simulink model "Commander_Stabilizer_Qdrone_serial"  (R2019a)
settings: Solver=ode2  StartTime=0.0  StopTime=inf  FixedStep=0.001  RelTol=1e-3  EnableMultiTasking=on
InitFcn:
  | set_param(gcs, 'ZoomFactor','FitSystem')
model workspace (MAT data in the model file):
  target_system = 1
undefined symbols (not defined in the file or in its folder): HIL, qc_get_step_size
libraries: quarc_library x53, simulink x24, simulink_extras x4
(part 1 of 4)
settings Model: SimulationMode=external  ExtModeTrigDuration=10000  Creator=dmadill  LastModifiedBy=user
settings SolverCC: PositivePriorityOrder=on
settings DataIOCC: LimitDataPoints=on  SaveFormat=Array  ReturnWorkspaceOutputs=off
settings OptimizationCC: LifeSpan=inf
settings DebuggingCC: SolverPrmCheckMsg=warning  SFUnexpectedBacktrackingDiag=warning  SFNoUnconditionalDefaultTransitionDiag=warning  SFExecutionAtInitializationDiag=none  ArithmeticOperatorsInVariantConditions=warning
settings HardwareCC: ProdBitPerLong=64  ProdLargestAtomicFloat=None  ProdHWDeviceType=Intel->x86-64
settings ModelReferenceCC: PropagateSignalLabelsOutOfModel=off
settings SFSimCC: SimUseLocalCustomCode=off
settings RTWCC: SystemTargetFile=quarc_linux_x64.tlc  TemplateMakefile=quarc_linux_x64_tmf  Description=QUARC Linux x64 Target  RTWUseLocalCustomCode=off
settings CodeAppCC: StateflowObjectComments=on
settings STFCustomTargetCC: TargetLibSuffix=.a  TargetPreCompLibLocation=C:\PROGRA~3\QUARC\lib\2019a\LINUX_~1\release  ConcurrentExecutionCompliant=on  SystemTargetFile=quarc_linux_x64.tlc
settings GRTTargetCC: TargetLibSuffix=.a  TargetPreCompLibLocation=C:\PROGRA~3\QUARC\lib\2019a\LINUX_~1\release  TargetLangStandard=C89/C90 (ANSI)  ParMdlRefBuildCompliant=off  CompOptLevelCompliant=off  CombineOutputUpdateFcns=off  MatFileLogging=off  CPPClassGenCompliant=off  GRTInterface=on  UseToolchainInfoCompliant=off  ExtMode=on  ExtModeMexFile=quarc_comm  ExtModeMexArgs='-w -d /tmp -uri %u -IP_address tcpip://192.168.1.157:18000', 'tcpip://192.168.1.25:17001?retries=10'
settings ConfigComp: CovMetricSettings=dw  CovHtmlReporting=on  CovSaveCumulativeToWorkspaceVar=on  CovSaveSingleToWorkspaceVar=on  CovExternalEMLEnable=off  CovSFcnEnable=off

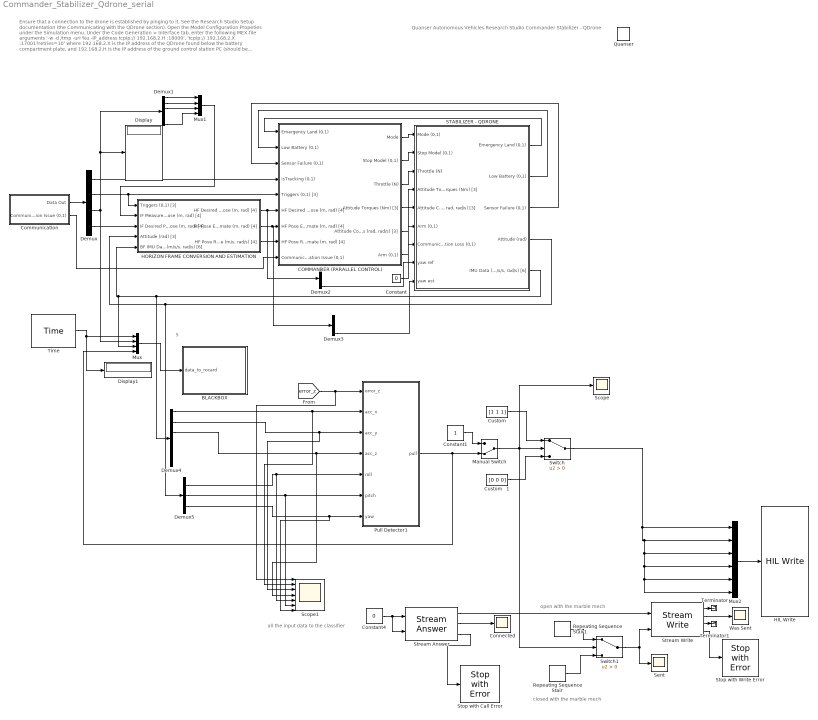
== system Commander_Stabilizer_Qdrone_serial ==
  note: all the input data to the classifier
  note: closed with the marble mech
  note: open with the marble mech
  note: Quanser Autonomous Vehicles Research Studio
      | Commander Stabilizer - QDrone
  note: Ensure that a connection to the drone is established by pinging to it. See the Research Studio Setup documentation (the Communicating with the QDrone section).
      | Open the Model Configuration Propeties under the Simulation menu.
      | Under the Code Generation > Interface tab, enter the following MEX-file arguments
      | '-w -d /tmp -uri %u -IP_address tcpip:// 192.168.2.H :18000', 'tcpip:// 192.168.2.X :17001?retries=10'
      | where 192.168.2.X is the IP address of the QDrone found below the battery compartment plate, and 192.168.2.H is the IP address of the ground control station PC (should be 192.168.2.5 by default).
      |
      | Under the QUARC menu, click on Build .
      |
      | Ensure that the Mission_Server_QDrone_Position_Control.slx model is running. If not, this model will stop immediately upon running. Click on Start under the QUARC menu.
      |
      | Ensure that the drone behaves as expected (see the steps in the Mission_Server_QDrone_Position_Control.slx model)
      | This model will automatically stop when the QDrone lands.
  note: 5
  "   Custom   " : Constant  Value=[1 1 1]
  "   Custom   1" : Constant  Value=[0 0 0]
  BLACKBOX : Subsystem
  COMMANDER (PARALLEL CONTROL) : Subsystem
  Communication : Subsystem
  Connected : Scope
  Constant : Constant  Value=0
  Constant1 : Constant
  Constant4 : Constant  Value=0
  Demux : Demux  Outputs=[1 3 6 4]
  Demux1 : Demux  Outputs=6
  Demux2 : Demux
  Demux3 : Demux
  Demux4 : Demux  Outputs=6
  Demux5 : Demux  Outputs=3
  Display : Display
  Display1 : Display
  HIL Write : quarc_library/Data Acquisition/Generic/Immediate I//O/HIL Write  object_name=HIL-1  analog_channels=[]  pwm_channels=[]  digital_channels=[5:7 9:23]  other_channels=[]  sample_time=-1  active=off  vector_input=on
      settings: SourceProductName=The database C:\Users\user\AppData\Roaming\MathWorks\MATLAB\R2017a\slblocks_master.db is locked, or a table in the database is locked. (database is locked)
  HORIZON FRAME CONVERSION AND ESTIMATION : Subsystem
  Manual Switch : ManualSwitch  CurrentSetting=0
  Mux : Mux  Inputs=[1 6 6 1]
  Mux1 : Mux
  Mux2 : Mux  Inputs=6
  Pull Detector1 : Subsystem
  Quanser : quarc_library/Logos/Quanser
  Repeating Sequence Stair : simulink/Sources/Repeating Sequence Stair  OutValues=[255 255 1 7 3 30 0 0 0 0 214].'  tsamp=-1  OutMin=[0]  OutMax=[]  OutDataTypeStr=fixdt(0,8,0)  OutputDataTypeScalingMode=Specify via dialog  OutDataType=fixdt(0,8,0)  ConRadixGroup=Best Precision: Vector-wise  OutScaling=[]
  Repeating Sequence Stair1 : simulink/Sources/Repeating Sequence Stair  OutValues=[255 255 1 7 3 30 32 3 0 0 179].'  tsamp=-1  OutMin=[0]  OutMax=[]  OutDataTypeStr=fixdt(0,8,0)  OutputDataTypeScalingMode=Specify via dialog  OutDataType=fixdt(0,8,0)  ConRadixGroup=Best Precision: Vector-wise  OutScaling=[]
  "STABILIZER - QDRONE " : Subsystem
  Scope : Scope
  Scope1 : Scope  NumInputPorts=7
  Sent : Scope
  Stop with Call Error : quarc_library/Sinks/Error Handling/Stop with Error  message_type=Interpret input as error code  message=Error occurred
      settings: SourceProductName=QUARC Targets
  Stop with Write Error : quarc_library/Sinks/Error Handling/Stop with Error  message_type=Interpret input as error code  message=Error occurred
      settings: SourceProductName=QUARC Targets
  Stream Answer : quarc_library/Communications/Intermediate/Stream Answer  uri_source=Specify via dialog (do not evaluate)  uri=serial://localhost:1?sndsize='16',baud='9600',word='8'  apply_uri_to_all_configs=on  send_buffer_size=128  receive_buffer_size=128  byte_order=little endian (Intel - LSB first)  sample_time=qc_get_step_size  active=off
      settings: AttributesFormatString="\"serial://localhost:1?sndsize='16',baud='9600',word='8'\""  SourceProductName=QUARC Targets
  Stream Write : quarc_library/Communications/Intermediate/Stream Write  optimization=Minimizing latency  send_dims=off
      settings: SourceProductName=QUARC Targets
  Switch : Switch  Criteria=u2 > Threshold
  Switch1 : Switch  Criteria=u2 > Threshold
  Terminator : Terminator
  Terminator1 : Terminator
  Time : quarc_library/Sources/Time/Time  time_source=Process CPU time  sample_time=qc_get_step_size
  Was Sent : Scope
  wires:
  COMMANDER (PARALLEL CONTROL)/2(Stop Model (0,1)) -> "STABILIZER - QDRONE "/2(Stop Model (0,1))
  "STABILIZER - QDRONE "/1(Emergency Land (0,1)) -> COMMANDER (PARALLEL CONTROL)/1(Emergency Land (0,1))
  COMMANDER (PARALLEL CONTROL)/4(Attitude Torques (Nm) [3]) -> "STABILIZER - QDRONE "/4(Attitude Torques (Nm) [3])
  Communication/1(Data Out) -> Demux/1
  Demux/2 -> COMMANDER (PARALLEL CONTROL)/5(Triggers (0,1) [3]), HORIZON FRAME CONVERSION AND ESTIMATION/1(Triggers (0,1) [3])
  "STABILIZER - QDRONE "/2(Low Battery (0,1)) -> COMMANDER (PARALLEL CONTROL)/2(Low Battery (0,1))
  "STABILIZER - QDRONE "/3(Sensor Failure (0,1)) -> COMMANDER (PARALLEL CONTROL)/3(Sensor Failure (0,1))
  COMMANDER (PARALLEL CONTROL)/6(Arm (0,1)) -> "STABILIZER - QDRONE "/6(Arm (0,1))
  COMMANDER (PARALLEL CONTROL)/3(Throttle (N)) -> "STABILIZER - QDRONE "/3(Throttle (N))
  Constant/1 -> "STABILIZER - QDRONE "/7(Communication Loss (0,1))
  COMMANDER (PARALLEL CONTROL)/5("Attitude Commands (rad, rad/s) [3]") -> "STABILIZER - QDRONE "/5("Attitude Commands (rad, rad, rad/s) [3]")
  COMMANDER (PARALLEL CONTROL)/1(Mode) -> "STABILIZER - QDRONE "/1(Mode (0,1))
  Communication/2(Communication Issue (0,1)) -> COMMANDER (PARALLEL CONTROL)/9(Communication Issue (0,1))
  "STABILIZER - QDRONE "/4(Attitude (rad)) -> Demux5/1, HORIZON FRAME CONVERSION AND ESTIMATION/4(Attitude (rad) [3])
  "STABILIZER - QDRONE "/5("IMU Data (m/s/s, rad/s) [6]") -> Demux4/1, Mux/3, HORIZON FRAME CONVERSION AND ESTIMATION/5("BF IMU Data (m/s/s, rad/s) [6]")
  HORIZON FRAME CONVERSION AND ESTIMATION/3("HF Pose Rate Estimate (m/s, rad/s) [4]") -> COMMANDER (PARALLEL CONTROL)/8("HF Pose Rate Estimate (m, rad) [4]")
  Demux/1 -> COMMANDER (PARALLEL CONTROL)/4(isTracking (0,1))
  Demux/4 -> HORIZON FRAME CONVERSION AND ESTIMATION/3("IF Desired Pose (m, rad) [4]")
  Demux/3 -> Demux1/1, Display/1, Mux/2
  Mux1/1 -> HORIZON FRAME CONVERSION AND ESTIMATION/2("IF Measured Pose (m, rad) [4]")
  Demux1/3 -> Mux1/3
  Demux1/6 -> Mux1/4
  Demux1/2 -> Mux1/2
  Demux1/1 -> Mux1/1
  Mux/1 -> BLACKBOX/1("data_to_rocard ")
  Time/1 -> Display1/1, Mux/1
  Demux2/4 -> "STABILIZER - QDRONE "/8(yaw ref)
  HORIZON FRAME CONVERSION AND ESTIMATION/1("HF Desired Pose (m, rad) [4]") -> Demux2/1, COMMANDER (PARALLEL CONTROL)/6("HF Desired Pose (m, rad) [4]")
  Demux3/4 -> "STABILIZER - QDRONE "/9(yaw est)
  HORIZON FRAME CONVERSION AND ESTIMATION/2("HF Pose Estimate (m, rad) [4]") -> Demux3/1, COMMANDER (PARALLEL CONTROL)/7("HF Pose Estimate (m, rad) [4]")
  Demux4/1 -> Pull Detector1/2(acc_x), Scope1/2
  Demux4/2 -> Pull Detector1/3(acc_y), Scope1/3
  Demux4/3 -> Pull Detector1/4(acc_z), Scope1/4
  [error_z] -> Scope1/1, Pull Detector1/1(error_z)
  Demux5/1 -> Pull Detector1/5(roll), Scope1/5
  Demux5/2 -> Pull Detector1/6(pitch), Scope1/6
  Demux5/3 -> Scope1/7, Pull Detector1/7(yaw)
  Mux2/1 -> HIL Write/1
  Switch/1 -> Mux2/6, Mux2/5, Mux2/4, Mux2/3, Mux2/2, Mux2/1
  Pull Detector1/1(pull) -> Mux/4, Manual Switch/2
  Manual Switch/1 -> Switch1/2, Switch/2, Scope/1
  "   Custom   "/1 -> Switch/1
  "   Custom   1"/1 -> Switch/3
  Constant1/1 -> Manual Switch/1
  Stream Write/4 -> Stop with Write Error/1
  Stream Answer/2 -> Connected/1
  Stream Write/3 -> Terminator1/1
  Stream Write/2 -> Was Sent/1
  Stream Answer/3 -> Stop with Call Error/1
  Stream Answer/1 -> Stream Write/1
  Switch1/1 -> Stream Write/2, Sent/1
  Constant4/1 -> Stream Answer/1, Stream Answer/2
  Stream Write/1 -> Terminator/1
  Repeating Sequence Stair1/1 -> Switch1/1
  Repeating Sequence Stair/1 -> Switch1/3

== system Commander_Stabilizer_Qdrone_serial/BLACKBOX ==
  "data_to_rocard " : Inport
  To Host File : quarc_library/Sinks/To Host/To Host File  file_name=saved_data/%m/record_data_%{date}_%{time}.mat  variable_name=optitack_imu_data  decimation=1  sample_time=-1  file_format=MAT-file v.5  options=No header or footer  append=off  final_file_name=saved_data/Commander_Stabilizer_Qdrone_serial/record_data_04-Apr-2021_22-18-28.mat  bitrate=2000000
  wires:
  "data_to_rocard "/1 -> To Host File/1

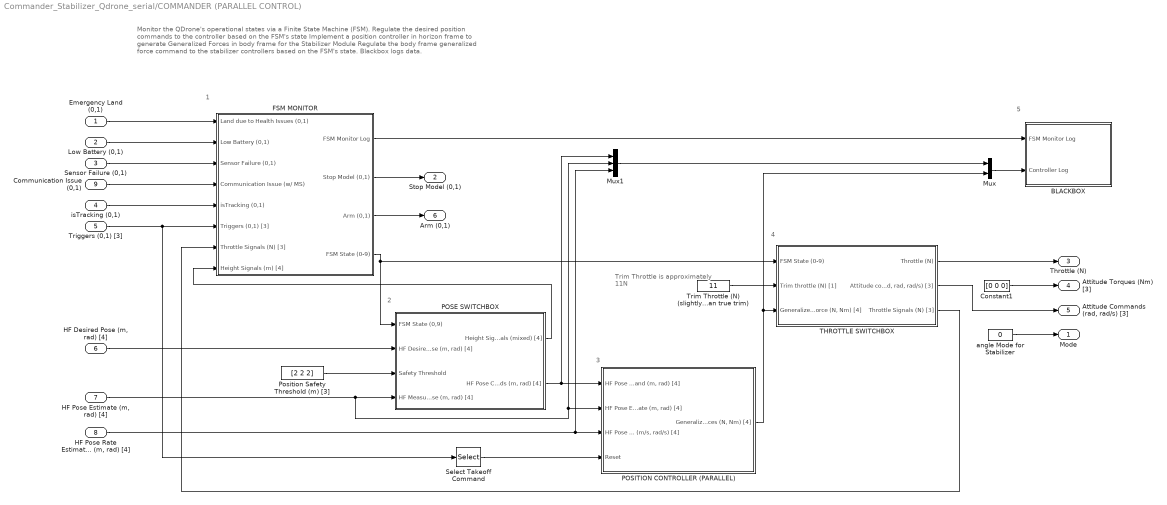
== system Commander_Stabilizer_Qdrone_serial/COMMANDER (PARALLEL CONTROL) ==
  note: 5
  note: 4
  note: 3
  note: 2
  note: 1
  note: Monitor the QDrone's operational states via a Finite State Machine (FSM).
      | Regulate the desired position commands to the controller based on the FSM's state
      | Implement a position controller in horizon frame to generate Generalized Forces in body frame for the Stabilizer Module
      | Regulate the body frame generalized force command to the stabilizer controllers based on the FSM's state.
      | Blackbox logs data.
  note: Trim Throttle is approximately 11N
  Emergency Land (0,1) : Inport
  Low Battery (0,1) : Inport  Port=2
  Sensor Failure (0,1) : Inport  Port=3
  isTracking (0,1) : Inport  Port=4
  Triggers (0,1) [3] : Inport  Port=5
  "HF Desired Pose (m, rad) [4]" : Inport  Port=6
  "HF Pose Estimate (m, rad) [4]" : Inport  Port=7
  "HF Pose Rate Estimate (m, rad) [4]" : Inport  Port=8
  Communication Issue (0,1) : Inport  Port=9
  BLACKBOX : Subsystem
  Constant1 : Constant  Value=[0 0 0]
  FSM MONITOR : Subsystem
  Mux : Mux  Inputs=2
  Mux1 : Mux  Inputs=3
  POSE SWITCHBOX : Subsystem
  POSITION CONTROLLER (PARALLEL) : Subsystem
  Position Safety Threshold (m) [3] : Constant  Value=[2 2 2]
  Select Takeoff Command : Selector  InputPortWidth=3  IndexOptions=Index vector (dialog)  Indices=[2]  OutputSizes=1
  "THROTTLE SWITCHBOX " : Subsystem
  Trim Throttle (N) (slightly lower than true trim) : Constant  Value=11
  angle Mode for Stabilizer : Constant  Value=0
  Mode : Outport
  Stop Model (0,1) : Outport  Port=2
  Throttle (N) : Outport  Port=3
  Attitude Torques (Nm) [3] : Outport  Port=4
  "Attitude Commands (rad, rad/s) [3]" : Outport  Port=5
  Arm (0,1) : Outport  Port=6
  wires:
  FSM MONITOR/1(FSM Monitor Log) -> BLACKBOX/1(FSM Monitor Log)
  FSM MONITOR/2(Stop Model (0,1)) -> Stop Model (0,1)/1
  FSM MONITOR/3(Arm (0,1)) -> Arm (0,1)/1
  Emergency Land (0,1)/1 -> FSM MONITOR/1(Land due to Health Issues (0,1))
  Low Battery (0,1)/1 -> FSM MONITOR/2(Low Battery (0,1))
  Sensor Failure (0,1)/1 -> FSM MONITOR/3(Sensor Failure (0,1))
  Communication Issue (0,1)/1 -> FSM MONITOR/4(Communication Issue (w/ MS))
  isTracking (0,1)/1 -> FSM MONITOR/5(isTracking (0,1))
  Select Takeoff Command/1 -> POSITION CONTROLLER (PARALLEL)/4(Reset)
  angle Mode for Stabilizer/1 -> Mode/1
  "HF Pose Estimate (m, rad) [4]"/1 -> Mux1/2, POSITION CONTROLLER (PARALLEL)/2("HF Pose Estimate (m, rad) [4]"), POSE SWITCHBOX/4("HF Measured Pose (m, rad) [4]")
  "HF Pose Rate Estimate (m, rad) [4]"/1 -> Mux1/3, POSITION CONTROLLER (PARALLEL)/3("HF Pose Rate (m/s, rad/s) [4]")
  Trim Throttle (N) (slightly lower than true trim)/1 -> "THROTTLE SWITCHBOX "/2(Trim throttle (N) [1])
  POSITION CONTROLLER (PARALLEL)/1("Generalized Forces (N, Nm) [4]") -> Mux/2, "THROTTLE SWITCHBOX "/3("Generalized Force (N, Nm) [4]")
  "HF Desired Pose (m, rad) [4]"/1 -> POSE SWITCHBOX/2("HF Desired Pose (m, rad) [4]")
  Position Safety Threshold (m) [3]/1 -> POSE SWITCHBOX/3(Safety Threshold)
  FSM MONITOR/4(FSM State (0-9)) -> POSE SWITCHBOX/1(FSM State (0,9)), "THROTTLE SWITCHBOX "/1(FSM State (0-9))
  "THROTTLE SWITCHBOX "/1(Throttle (N)) -> Throttle (N)/1
  POSE SWITCHBOX/1(Height Signals (mixed) [4]) -> FSM MONITOR/8(Height Signals (m) [4])
  "THROTTLE SWITCHBOX "/3(Throttle Signals (N) [3]) -> FSM MONITOR/7(Throttle Signals (N) [3])
  Triggers (0,1) [3]/1 -> FSM MONITOR/6(Triggers (0,1) [3]), Select Takeoff Command/1
  Mux/1 -> BLACKBOX/2(Controller Log)
  POSE SWITCHBOX/2("HF Pose Commands (m, rad) [4]") -> Mux1/1, POSITION CONTROLLER (PARALLEL)/1("HF Pose Command (m, rad) [4]")
  Mux1/1 -> Mux/1
  Constant1/1 -> Attitude Torques (Nm) [3]/1
  "THROTTLE SWITCHBOX "/2("Attitude commands (rad, rad, rad/s) [3]") -> "Attitude Commands (rad, rad/s) [3]"/1

== system Commander_Stabilizer_Qdrone_serial/Communication ==
  note: Argument (- IP_address ) is set at the MEX-file arguments found at Model Configuration Properties > Code Generation > Interface
      |
      | Format:
      | tcpip://192.168.2.H:18000
      | where H is the last digits of your ground station's IP address (use ipconfig in a command prompt to find it out).
  Constant : Constant
  Detect Communication Loss : Subsystem
  Display : Display
  Memory : Memory  InheritSampleTime=on  LinearizeMemory=on  LinearizeAsDelay=on
  Model Argument : quarc_library/Sources/Signals/Model Argument  argument_name=IP_address  has_value=on  data_type_mode=Specify via dialog  data_type=char  max_length=80  variable_size=off
      settings: AttributesFormatString=(-%<argument_name>)  SourceProductName=QUARC Targets
  Select Timestamp received and send back immediately (for calculating loopback time) : Selector  InputPortWidth=15  IndexOptions=Index vector (dialog)  Indices=[15]  OutputSizes=1
  Select the rest of the data : Selector  InputPortWidth=15  IndexOptions=Index vector (dialog)  Indices=[1:14]  OutputSizes=1
  Stream Client : quarc_library/Communications/Basic/Stream Client  uri_source=External input port  uri=tcpip://192.168.2.3:18669  apply_uri_to_all_configs=on  send_buffer_size=1460  receive_buffer_size=1460  byte_order=little endian (Intel - LSB first)  optimization=Minimum latency  send_options=Send most recent data  receive_options=Receive most recent data  default_value=zeros(1,15)  sample_time=qc_get_step_size  active=off  implementation=Use blocking I/O in a separate thread  send_fifo_size=1000  receive_fifo_size=1000  send_priority=0  receive_priority=0  send_dimensions=off  receive_dimensions=off  max_dimensions=-1  data_type=Inherited via back propagation  type_expr=BusObject
  String Display : quarc_library/Strings/String Display  alignment=center  display_mode=Single line  sample_time=-1
      settings: SourceProductName=QUARC Targets
  Terminator1 : Terminator
  Terminator2 : Terminator
  Data Out : Outport
  Communication Issue (0,1) : Outport  Port=2
  wires:
  Stream Client/5 -> Terminator2/1
  Model Argument/1 -> Stream Client/3, String Display/1
  Constant/1 -> Stream Client/2
  Stream Client/3 -> Terminator1/1
  Stream Client/4 -> Detect Communication Loss/3(Data Out), Select Timestamp received and send back immediately (for calculating loopback time)/1, Select the rest of the data/1
  Memory/1 -> Stream Client/1
  Stream Client/1 -> Detect Communication Loss/1(State)
  Stream Client/2 -> Detect Communication Loss/2(Error)
  Detect Communication Loss/1(Communication Issue) -> Communication Issue (0,1)/1
  Select the rest of the data/1 -> Data Out/1
  Select Timestamp received and send back immediately (for calculating loopback time)/1 -> Display/1, Memory/1

== system Commander_Stabilizer_Qdrone_serial/HORIZON FRAME CONVERSION AND ESTIMATION ==
  note: IF => Inertial Frame
      | BF => Body Frame
      | HF => Horizon Frame
  note: 6
  note: 5
  note: 4
  note: 3
  note: 2
  note: 1
  note: Steps:
      |
      | Estimate the Yaw Angle from the gyroscopic yaw rate signal and the localization yaw correction signal.
      | Use this yaw estimate, along with the roll/pitch estimates from the stabilizer to calculate the rotation matrices that convert data from the Body and Inertial Frames to the Horizon frame, where position control takes place
      | Transform Body Frame Net Accelerations (from accelerometer) to Horizon Frame Vehicle Accelerations
      | Transform Inertial Frame Desired and Measured Positions to the Horizon Frame Pose Commands and Estimates respectively
      | Calculate the Pose Rate Estimates
      | Saturate and Rate Limit the IF Desired Pose based on workspace limitations
  Triggers (0,1) [3] : Inport
  "IF Measured Pose (m, rad) [4]" : Inport  Port=2
  "IF Desired Pose (m, rad) [4]" : Inport  Port=3
  Attitude (rad) [3] : Inport  Port=4
  "BF IMU Data (m/s/s, rad/s) [6]" : Inport  Port=5
  Calculate Rotation Matrices : Subsystem
  Estimate Yaw Angle : Subsystem
  Pitch : Selector  InputPortWidth=3  IndexOptions=Index vector (dialog)  Indices=[2]  OutputSizes=1
  Pose Rate Estimation : Subsystem
  Rate Limiter : RateLimiter  RisingSlewLimit=[2 2 3 2]  FallingSlewLimit=[-2 -2 -3 -2]  SampleTimeMode=inherited  InitialCondition=[0 0 0 0]
  Roll : Selector  InputPortWidth=3  IndexOptions=Index vector (dialog)  Indices=[1]  OutputSizes=1
  Saturation : Saturate  UpperLimit=[2.5 2.5 3 Inf]  LowerLimit=[-2.5 -2.5 0 -Inf]
  Select Gyro Yaw Rate (rad/s) : Selector  InputPortWidth=6  IndexOptions=Index vector (dialog)  Indices=[6]  OutputSizes=1
  Select Linear Acceleration : Selector  InputPortWidth=6  IndexOptions=Index vector (dialog)  Indices=[1 2 3]  OutputSizes=1
  Select Takeoff Command : Selector  InputPortWidth=3  IndexOptions=Index vector (dialog)  Indices=[2]  OutputSizes=1
  Select Yaw Estimate : Selector  InputPortWidth=4  IndexOptions=Index vector (dialog)  Indices=4  OutputSizes=1
  Transform from Body Frame to Horizon Frame : Subsystem
  Transform from Inertial Frame to Horizon Frame : Subsystem
  "HF Desired Pose (m, rad) [4]" : Outport
  "HF Pose Estimate (m, rad) [4]" : Outport  Port=2
  "HF Pose Rate Estimate (m/s, rad/s) [4]" : Outport  Port=3
  wires:
  "BF IMU Data (m/s/s, rad/s) [6]"/1 -> Select Linear Acceleration/1, Select Gyro Yaw Rate (rad/s)/1
  Select Gyro Yaw Rate (rad/s)/1 -> Estimate Yaw Angle/1(Yaw Rate (rad/s)), Pose Rate Estimation/3(Yaw Rate (rad/s))  "Gyroscope Yaw Rate (rad/s)"
  "IF Measured Pose (m, rad) [4]"/1 -> Transform from Inertial Frame to Horizon Frame/4("IF Pose Measurement (m, rad) [4]"), Select Yaw Estimate/1
  Estimate Yaw Angle/1(Yaw Estimate (rad)) -> Transform from Inertial Frame to Horizon Frame/3(Yaw Estimate), Calculate Rotation Matrices/3(Yaw Estimate (rad))
  Select Yaw Estimate/1 -> Estimate Yaw Angle/2(Yaw Correction (rad))
  Triggers (0,1) [3]/1 -> Select Takeoff Command/1
  Attitude (rad) [3]/1 -> Pitch/1, Roll/1
  Roll/1 -> Calculate Rotation Matrices/1(" Roll Estimate (rad)")
  Pitch/1 -> Calculate Rotation Matrices/2(Pitch Estimate (rad))
  Pose Rate Estimation/1("HF Pose Rate Estimate (m/s, rad/s) [4]") -> "HF Pose Rate Estimate (m/s, rad/s) [4]"/1
  Transform from Inertial Frame to Horizon Frame/1("HF Pose Estimate (m, rad) [4]") -> "HF Pose Estimate (m, rad) [4]"/1, Pose Rate Estimation/2("HF Pose Measurement (m, rad) [4]")
  Calculate Rotation Matrices/2(HF_R_IF) -> Transform from Inertial Frame to Horizon Frame/1(HF_R_IF)
  "IF Desired Pose (m, rad) [4]"/1 -> Saturation/1
  Transform from Inertial Frame to Horizon Frame/2("HF Pose Command (m, rad) [4]") -> "HF Desired Pose (m, rad) [4]"/1
  Calculate Rotation Matrices/1(HF_R_BF) -> Transform from Body Frame to Horizon Frame/1(HF_R_BF)
  Select Linear Acceleration/1 -> Transform from Body Frame to Horizon Frame/2(BF Net Acceleration (m/s/s) [3])  "BF Net Acceleration"
  Transform from Body Frame to Horizon Frame/1(HF Vehicle Acceleration (m/s/s) [3]) -> Pose Rate Estimation/1(HF Vehicle Acceleration (m/s/s) [3])
  Select Takeoff Command/1 -> Estimate Yaw Angle/3(Reset), Pose Rate Estimation/4(Reset)  "Reset Condition"
  Rate Limiter/1 -> Transform from Inertial Frame to Horizon Frame/2("IF Pose Command (m, rad) [4]")
  Saturation/1 -> Rate Limiter/1

== system Commander_Stabilizer_Qdrone_serial/Pull Detector1 ==
  error_z : Inport
  acc_x : Inport  Port=2
  acc_y : Inport  Port=3
  acc_z : Inport  Port=4
  roll : Inport  Port=5
  pitch : Inport  Port=6
  yaw : Inport  Port=7
  Constant : Constant  Value=50  OutDataTypeStr=single
  MATLAB Function : MATLAB Function  TreatAsAtomicUnit=on
  MATLAB Function1 : MATLAB Function  TreatAsAtomicUnit=on
  Scope4 : Scope  NumInputPorts=3
  pull : Outport  VectorParamsAs1DForOutWhenUnconnected=on
  wires:
  yaw/1 -> MATLAB Function/7(yaw)
  roll/1 -> MATLAB Function/5(roll)
  Constant/1 -> MATLAB Function1/2(threshold)
  acc_x/1 -> MATLAB Function/2(acc_x)
  acc_y/1 -> MATLAB Function/3(acc_y)
  MATLAB Function/1(detection_output) -> MATLAB Function1/1(u), Scope4/1
  acc_z/1 -> MATLAB Function/4(acc_z)
  pitch/1 -> MATLAB Function/6(pitch)
  error_z/1 -> Scope4/3, MATLAB Function/1(error_z)
  MATLAB Function1/1(y) -> Scope4/2, pull/1

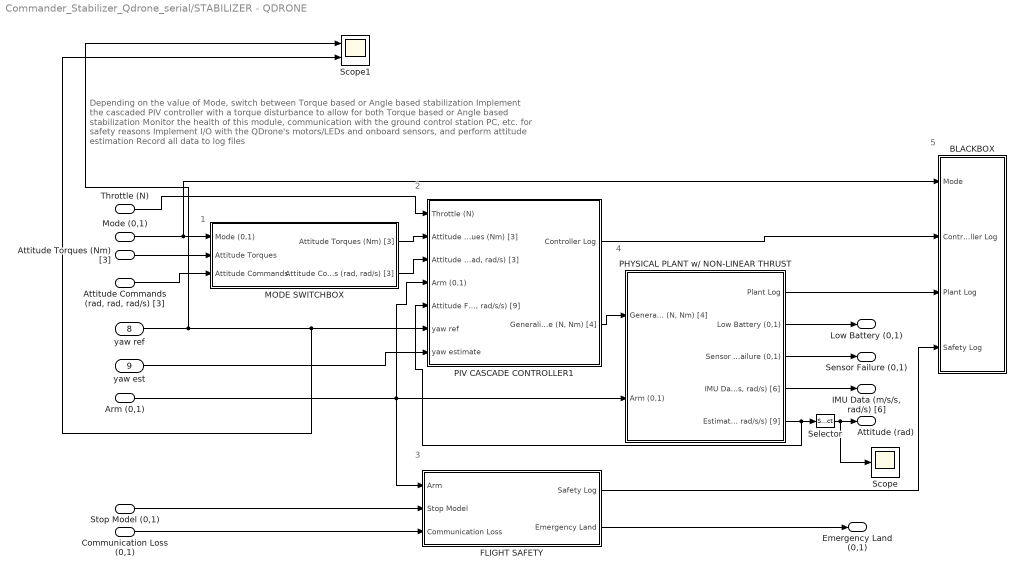
== system Commander_Stabilizer_Qdrone_serial/STABILIZER - QDRONE  ==
  note: 5
  note: 4
  note: 3
  note: 2
  note: 1
  note: Depending on the value of Mode, switch between Torque based or Angle based stabilization
      | Implement the cascaded PIV controller with a torque disturbance to allow for both Torque based or Angle based stabilization
      | Monitor the health of this module, communication with the ground control station PC, etc. for safety reasons
      | Implement I/O with the QDrone's motors/LEDs and onboard sensors, and perform attitude estimation
      | Record all data to log files
  Mode (0,1) : Inport
  Stop Model (0,1) : Inport  Port=2
  Throttle (N) : Inport  Port=3
  Attitude Torques (Nm) [3] : Inport  Port=4
  "Attitude Commands (rad, rad, rad/s) [3]" : Inport  Port=5
  Arm (0,1) : Inport  Port=6
  Communication Loss (0,1) : Inport  Port=7
  yaw ref : Inport  Port=8
  yaw est : Inport  Port=9
  BLACKBOX : Subsystem
  FLIGHT SAFETY : Subsystem
  MODE SWITCHBOX : Subsystem
  PHYSICAL PLANT w/ NON-LINEAR THRUST : Subsystem
  PIV CASCADE CONTROLLER1 : Subsystem
  Scope : Scope
  Scope1 : Scope  NumInputPorts=2
  Selector : Selector  InputPortWidth=9  IndexOptions=Index vector (dialog)  Indices=[1:3]  OutputSizes=1
  Emergency Land (0,1) : Outport
  Low Battery (0,1) : Outport  Port=2
  Sensor Failure (0,1) : Outport  Port=3
  Attitude (rad) : Outport  Port=4
  "IMU Data (m/s/s, rad/s) [6]" : Outport  Port=5
  wires:
  PIV CASCADE CONTROLLER1/1(Controller Log) -> BLACKBOX/2(Controller Log)
  Attitude Torques (Nm) [3]/1 -> MODE SWITCHBOX/2(Attitude Torques)
  PHYSICAL PLANT w/ NON-LINEAR THRUST/1(Plant Log) -> BLACKBOX/3(Plant Log)
  FLIGHT SAFETY/1(Safety Log) -> BLACKBOX/4(Safety Log)
  PHYSICAL PLANT w/ NON-LINEAR THRUST/5("Estimated Attitude (rad, rad/s, rad/s/s) [9]") -> PIV CASCADE CONTROLLER1/5("Attitude Feedback (rad, rad/s, rad/s/s) [9]"), Selector/1
  FLIGHT SAFETY/2(Emergency Land) -> Emergency Land (0,1)/1
  PIV CASCADE CONTROLLER1/2("Generalized Force (N, Nm) [4]") -> PHYSICAL PLANT w/ NON-LINEAR THRUST/1("Generalized Force (N, Nm) [4]")
  PHYSICAL PLANT w/ NON-LINEAR THRUST/2(Low Battery (0,1)) -> Low Battery (0,1)/1
  Stop Model (0,1)/1 -> FLIGHT SAFETY/2(Stop Model)
  Arm (0,1)/1 -> PIV CASCADE CONTROLLER1/4(Arm (0,1)), PHYSICAL PLANT w/ NON-LINEAR THRUST/2(Arm (0,1)), FLIGHT SAFETY/1(Arm)
  Communication Loss (0,1)/1 -> FLIGHT SAFETY/3(Communication Loss)
  PHYSICAL PLANT w/ NON-LINEAR THRUST/3(Sensor Failure (0,1)) -> Sensor Failure (0,1)/1
  PHYSICAL PLANT w/ NON-LINEAR THRUST/4("IMU Data (m/s/s, rad/s) [6]") -> "IMU Data (m/s/s, rad/s) [6]"/1
  Throttle (N)/1 -> PIV CASCADE CONTROLLER1/1(Throttle (N))
  "Attitude Commands (rad, rad, rad/s) [3]"/1 -> MODE SWITCHBOX/3(Attitude Commands)
  Mode (0,1)/1 -> BLACKBOX/1(Mode), MODE SWITCHBOX/1(Mode (0,1))
  MODE SWITCHBOX/2("Attitude Commands (rad, rad/s) [3]") -> PIV CASCADE CONTROLLER1/3("Attitude Commands (rad, rad, rad/s) [3]")
  MODE SWITCHBOX/1(Attitude Torques (Nm) [3]) -> PIV CASCADE CONTROLLER1/2(Attitude Torques (Nm) [3])
  Selector/1 -> Scope/1, Attitude (rad)/1
  yaw est/1 -> PIV CASCADE CONTROLLER1/7("yaw estimate ")
  yaw ref/1 -> Scope1/2, PIV CASCADE CONTROLLER1/6("yaw ref "), Scope1/1

== system Commander_Stabilizer_Qdrone_serial/COMMANDER (PARALLEL CONTROL)/BLACKBOX ==
  FSM Monitor Log : Inport
  Controller Log : Inport  Port=2
  Mux : Mux  Inputs=2
  To Host File : quarc_library/Sinks/To Host/To Host File  file_name=saved_data/%m/Commander_%{date}_%{time}.mat  variable_name=commander_data  decimation=1  sample_time=-1  file_format=MAT-file v.5  options=No header or footer  append=off  final_file_name=saved_data/Commander_Stabilizer_Qdrone_serial/Commander_04-Apr-2021_22-18-28.mat  bitrate=2000000
  wires:
  Mux/1 -> To Host File/1
  FSM Monitor Log/1 -> Mux/1
  Controller Log/1 -> Mux/2

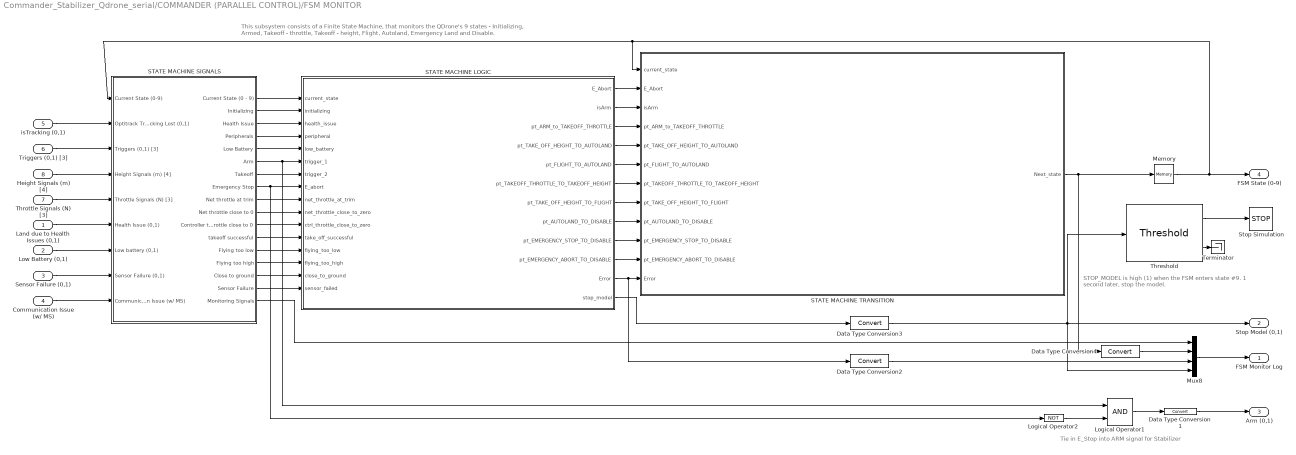
== system Commander_Stabilizer_Qdrone_serial/COMMANDER (PARALLEL CONTROL)/FSM MONITOR ==
  note: This subsystem consists of a Finite State Machine, that monitors the QDrone's 9 states - Initializing, Armed, Takeoff - throttle, Takeoff - height, Flight, Autoland, Emergency Land and Disable.
  note: Tie in E_Stop into ARM signal for Stabilizer
  note: STOP_MODEL is high (1) when the FSM enters state #9.
      | 1 second later, stop the model.
  Land due to Health Issues (0,1) : Inport
  Low Battery (0,1) : Inport  Port=2
  Sensor Failure (0,1) : Inport  Port=3
  Communication Issue (w/ MS) : Inport  Port=4
  isTracking (0,1) : Inport  Port=5
  Triggers (0,1) [3] : Inport  Port=6
  Throttle Signals (N) [3] : Inport  Port=7
  Height Signals (m) [4] : Inport  Port=8
  Data Type Conversion{1..4} (4 alike) : DataTypeConversion
  Logical Operator1 : Logic  AllPortsSameDT=off  OutDataTypeStr=boolean
  Logical Operator2 : Logic  Operator=NOT  AllPortsSameDT=off  OutDataTypeStr=boolean
  Memory : Memory  InitialCondition=1
  Mux8 : Mux  Inputs=[17 1 1 1]
  STATE MACHINE LOGIC : MATLAB Function  TreatAsAtomicUnit=on
  STATE MACHINE SIGNALS : Subsystem
  STATE MACHINE TRANSITION : MATLAB Function  TreatAsAtomicUnit=on
  Stop Simulation : Stop
  Terminator : Terminator
  Threshold : quarc_library/Discontinuities/Threshold  operator=>=  param_src=Specify via dialog  threshold=0.5  duration=1
      settings: SourceProductName=QUARC Targets
  FSM Monitor Log : Outport
  Stop Model (0,1) : Outport  Port=2
  Arm (0,1) : Outport  Port=3
  FSM State (0-9) : Outport  Port=4
  wires:
  STATE MACHINE LOGIC/1(E_Abort) -> STATE MACHINE TRANSITION/2(E_Abort)
  STATE MACHINE LOGIC/11(Error) -> STATE MACHINE TRANSITION/12(Error), Data Type Conversion2/1
  STATE MACHINE LOGIC/6(pt_TAKEOFF_THROTTLE_TO_TAKEOFF_HEIGHT) -> STATE MACHINE TRANSITION/7(pt_TAKEOFF_THROTTLE_TO_TAKEOFF_HEIGHT)
  STATE MACHINE LOGIC/7(pt_TAKE_OFF_HEIGHT_TO_FLIGHT) -> STATE MACHINE TRANSITION/8(pt_TAKE_OFF_HEIGHT_TO_FLIGHT)
  STATE MACHINE LOGIC/8(pt_AUTOLAND_TO_DISABLE) -> STATE MACHINE TRANSITION/9(pt_AUTOLAND_TO_DISABLE)
  STATE MACHINE LOGIC/9(pt_EMERGENCY_STOP_TO_DISABLE) -> STATE MACHINE TRANSITION/10(pt_EMERGENCY_STOP_TO_DISABLE)
  STATE MACHINE LOGIC/10(pt_EMERGENCY_ABORT_TO_DISABLE) -> STATE MACHINE TRANSITION/11(pt_EMERGENCY_ABORT_TO_DISABLE)
  STATE MACHINE SIGNALS/2(Initializing) -> STATE MACHINE LOGIC/2(initializing)
  STATE MACHINE SIGNALS/3(Health Issue) -> STATE MACHINE LOGIC/3(health_issue)
  STATE MACHINE SIGNALS/4(Peripherals) -> STATE MACHINE LOGIC/4(peripheral)
  STATE MACHINE SIGNALS/5(Low Battery) -> STATE MACHINE LOGIC/5(low_battery)
  STATE MACHINE SIGNALS/7(Takeoff) -> STATE MACHINE LOGIC/7(trigger_2)
  STATE MACHINE SIGNALS/9(Net throttle at trim) -> STATE MACHINE LOGIC/9(net_throttle_at_trim)
  STATE MACHINE SIGNALS/10(Net throttle close to 0) -> STATE MACHINE LOGIC/10(net_throttle_close_to_zero)
  STATE MACHINE SIGNALS/11(Controller throttle close to 0) -> STATE MACHINE LOGIC/11(ctrl_throttle_close_to_zero)
  STATE MACHINE SIGNALS/12(takeoff successful) -> STATE MACHINE LOGIC/12(take_off_successful)
  STATE MACHINE SIGNALS/13(Flying too low) -> STATE MACHINE LOGIC/13(flying_too_low)
  STATE MACHINE SIGNALS/14(Flying too high) -> STATE MACHINE LOGIC/14(flying_too_high)
  STATE MACHINE SIGNALS/15(Close to ground) -> STATE MACHINE LOGIC/15(close_to_ground)
  STATE MACHINE TRANSITION/1(Next_state) -> Data Type Conversion4/1, Memory/1
  Mux8/1 -> FSM Monitor Log/1
  STATE MACHINE SIGNALS/1("Current State (0 - 9)  ") -> STATE MACHINE LOGIC/1(current_state)
  STATE MACHINE SIGNALS/16("  Sensor Failure") -> STATE MACHINE LOGIC/16(sensor_failed)
  STATE MACHINE SIGNALS/17(Monitoring Signals) -> Mux8/1
  Sensor Failure (0,1)/1 -> STATE MACHINE SIGNALS/8(Sensor Failure (0,1))
  Low Battery (0,1)/1 -> STATE MACHINE SIGNALS/7(Low battery (0,1))
  Land due to Health Issues (0,1)/1 -> STATE MACHINE SIGNALS/6("Health Issue (0,1)  ")
  Data Type Conversion1/1 -> Arm (0,1)/1
  Logical Operator1/1 -> Data Type Conversion1/1
  STATE MACHINE SIGNALS/8(Emergency Stop) -> Logical Operator2/1, STATE MACHINE LOGIC/8(E_abort)
  Logical Operator2/1 -> Logical Operator1/2
  STATE MACHINE SIGNALS/6(Arm) -> Logical Operator1/1, STATE MACHINE LOGIC/6(trigger_1)
  Triggers (0,1) [3]/1 -> STATE MACHINE SIGNALS/3(Triggers (0,1) [3])
  Communication Issue (w/ MS)/1 -> STATE MACHINE SIGNALS/9(Communication Issue (w/ MS))
  isTracking (0,1)/1 -> STATE MACHINE SIGNALS/2("Optitrack Tracking Lost (0,1)  ")
  Data Type Conversion2/1 -> Mux8/3
  Data Type Conversion4/1 -> Mux8/2
  Throttle Signals (N) [3]/1 -> STATE MACHINE SIGNALS/5(Throttle Signals (N) [3])
  Height Signals (m) [4]/1 -> STATE MACHINE SIGNALS/4(Height Signals (m) [4])
  Threshold/2 -> Terminator/1
  Data Type Conversion3/1 -> Threshold/1, Stop Model (0,1)/1, Mux8/4
  Threshold/1 -> Stop Simulation/1
  Memory/1 -> FSM State (0-9)/1, STATE MACHINE TRANSITION/1(current_state), STATE MACHINE SIGNALS/1(Current State (0-9))
  STATE MACHINE LOGIC/2(isArm) -> STATE MACHINE TRANSITION/3(isArm)
  STATE MACHINE LOGIC/3(pt_ARM_to_TAKEOFF_THROTTLE) -> STATE MACHINE TRANSITION/4(pt_ARM_to_TAKEOFF_THROTTLE)
  STATE MACHINE LOGIC/4(pt_TAKE_OFF_HEIGHT_TO_AUTOLAND) -> STATE MACHINE TRANSITION/5(pt_TAKE_OFF_HEIGHT_TO_AUTOLAND)
  STATE MACHINE LOGIC/5(pt_FLIGHT_TO_AUTOLAND) -> STATE MACHINE TRANSITION/6(pt_FLIGHT_TO_AUTOLAND)
  STATE MACHINE LOGIC/12(stop_model) -> Data Type Conversion3/1

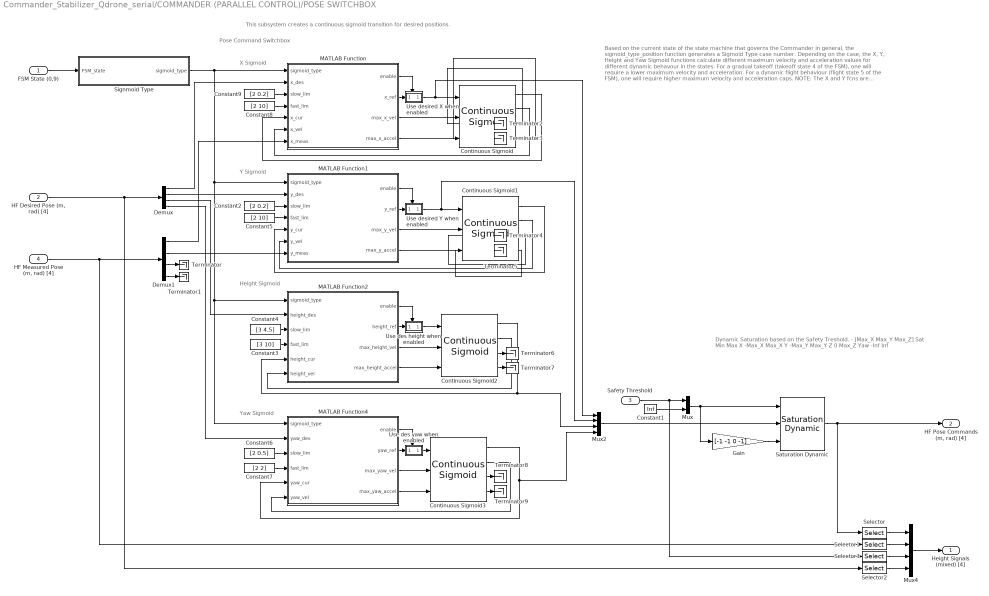
== system Commander_Stabilizer_Qdrone_serial/COMMANDER (PARALLEL CONTROL)/POSE SWITCHBOX ==
  note: Dynamic Saturation based on the Safety Treshold. - [Max_X Max_Y Max_Z]
      |
      | Sat Min Max
      | X -Max_X Max_X
      | Y -Max_Y Max_Y
      | Z 0 Max_Z
      | Yaw -Inf Inf
  note: Based on the current state of the state machine that governs the Commander in general,
      | the sigmoid_type_position function generates a Sigmoid Type case number. Depending on
      | the case, the X, Y, Height and Yaw Sigmoid functions calculate different maximum velocity
      | and acceleration values for different dynamic behavour in the states.
      |
      | For a gradual takeoff (takeoff state 4 of the FSM), one will require a lower maximum velocity
      | and acceleration. For a dynamic flight behaviour (flight state 5 of the FSM), one will require
      | higher maximum velocity and acceleration caps.
      |
      | NOTE: The X and Y fcns are logically identical due to the generally symmetric X and Y behaviour.
      | The Z and Yaw fcns are different.
  note: This subsystem creates a continuous sigmoid transition for desired positions.
  note: Height Sigmoid
  note: Pose Command Switchbox
  note: X Sigmoid
  note: Yaw Sigmoid
  note: Y Sigmoid
  FSM State (0,9) : Inport
  "HF Desired Pose (m, rad) [4]" : Inport  Port=2
  Safety Threshold : Inport  Port=3
  "HF Measured Pose (m, rad) [4]" : Inport  Port=4
  Constant1 : Constant  Value=Inf
  Constant2 : Constant  Value=[2 0.2]
  Constant3 : Constant  Value=[3 10]
  Constant4 : Constant  Value=[3 4.5]
  Constant5 : Constant  Value=[2 10]
  Constant6 : Constant  Value=[2 0.5]
  Constant7 : Constant  Value=[2 2]
  Constant8 : Constant  Value=[2 10]
  Constant9 : Constant  Value=[2 0.2]
  Continuous Sigmoid{,1..3} (4 alike) : quarc_library/Sources/Sigmoids/Continuous Sigmoid  params_source=External (input ports)  max_velocity=2  max_acceleration=10  initial_position=0  initial_velocity=0  hold_off=0.5  input_sample_time=-1  output_sample_time=qc_get_step_size
      settings: SourceProductName=QUARC Targets
  Demux : Demux
  Demux1 : Demux
  Gain : Gain  Gain=[-1 -1 0 -1]
  MATLAB Function : MATLAB Function  TreatAsAtomicUnit=on
  MATLAB Function1 : MATLAB Function  TreatAsAtomicUnit=on
  MATLAB Function2 : MATLAB Function  TreatAsAtomicUnit=on
  MATLAB Function4 : MATLAB Function  TreatAsAtomicUnit=on
  Mux : Mux  Inputs=2
  Mux2 : Mux
  Mux4 : Mux
  Saturation Dynamic : simulink/Discontinuities/Saturation Dynamic  OutMin=[]  OutMax=[]  OutDataTypeStr=Inherit: Same as second input  OutDataType=fixdt(1, 16)  OutScaling=2^-10  DoSatur=off
  Selector : Selector  InputPortWidth=4  IndexOptions=Index vector (dialog)  Indices=[3]  OutputSizes=1
  Selector1 : Selector  InputPortWidth=4  IndexOptions=Index vector (dialog)  Indices=[3]  OutputSizes=1
  Selector2 : Selector  InputPortWidth=4  IndexOptions=Index vector (dialog)  Indices=[3]  OutputSizes=1
  Selector3 : Selector  InputPortWidth=3  IndexOptions=Index vector (dialog)  Indices=[3]  OutputSizes=1
  Signmoid Type : MATLAB Function  TreatAsAtomicUnit=on
  Terminator{,1..9} (10 alike) : Terminator
  Use des height when enabled : Subsystem  TreatAsAtomicUnit=on
  Use des yaw when enabled : Subsystem  TreatAsAtomicUnit=on
  Use desired X when enabled : Subsystem  TreatAsAtomicUnit=on
  Use desired Y when enabled : Subsystem  TreatAsAtomicUnit=on
  Height Signals (mixed) [4] : Outport
  "HF Pose Commands (m, rad) [4]" : Outport  Port=2
  wires:
  Selector/1 -> Mux4/1
  Selector1/1 -> Mux4/2
  Selector2/1 -> Mux4/4
  Selector3/1 -> Mux4/3
  Safety Threshold/1 -> Mux/1, Selector3/1
  Mux/1 -> Saturation Dynamic/1, Gain/1
  Constant1/1 -> Mux/2
  Saturation Dynamic/1 -> "HF Pose Commands (m, rad) [4]"/1, Selector/1
  Mux2/1 -> Saturation Dynamic/2
  Mux4/1 -> Height Signals (mixed) [4]/1
  Gain/1 -> Saturation Dynamic/3
  Demux/2 -> MATLAB Function1/2(y_des)
  Constant4/1 -> MATLAB Function2/3(slow_lim)
  Use desired Y when enabled/1(Out1) -> Mux2/2, Continuous Sigmoid1/1
  MATLAB Function2/3(max_height_vel) -> Continuous Sigmoid2/2
  Continuous Sigmoid3/3 -> Terminator8/1
  Demux1/4 -> Terminator1/1
  MATLAB Function4/1(enable) -> Use des yaw when enabled/Enable
  Use des yaw when enabled/1(Out1) -> Continuous Sigmoid3/1
  Constant5/1 -> MATLAB Function1/4(fast_lim)
  Continuous Sigmoid1/2 -> MATLAB Function1/6(y_vel)
  Constant2/1 -> MATLAB Function1/3(slow_lim)
  Constant6/1 -> MATLAB Function4/3(slow_lim)
  Demux1/1 -> MATLAB Function/7(x_meas)
  MATLAB Function1/2(y_ref) -> Use desired Y when enabled/1(h_d (m) [1])
  Demux/3 -> MATLAB Function2/2(height_des)
  Constant7/1 -> MATLAB Function4/4(fast_lim)
  Continuous Sigmoid1/4 -> Terminator5/1
  MATLAB Function1/1(enable) -> Use desired Y when enabled/Enable
  Continuous Sigmoid2/4 -> Terminator7/1
  Demux1/3 -> Terminator/1
  Signmoid Type/1(sigmoid_type) -> MATLAB Function4/1(sigmoid_type), MATLAB Function2/1(sigmoid_type), MATLAB Function1/1(sigmoid_type), MATLAB Function/1(sigmoid_type)
  MATLAB Function/3(max_x_vel) -> Continuous Sigmoid/2
  MATLAB Function2/1(enable) -> Use des height when enabled/Enable
  Constant9/1 -> MATLAB Function/3(slow_lim)
  Continuous Sigmoid2/2 -> MATLAB Function2/6(height_vel)
  Continuous Sigmoid1/1 -> MATLAB Function1/5(y_cur)
  MATLAB Function4/4(max_yaw_accel) -> Continuous Sigmoid3/3
  Demux/1 -> MATLAB Function/2(x_des)
  Constant8/1 -> MATLAB Function/4(fast_lim)
  MATLAB Function1/3(max_y_vel) -> Continuous Sigmoid1/2
  Continuous Sigmoid3/2 -> MATLAB Function4/6(yaw_vel)
  MATLAB Function2/2(height_ref) -> Use des height when enabled/1(h_d (m) [1])
  MATLAB Function/4(max_x_accel) -> Continuous Sigmoid/3
  Continuous Sigmoid2/3 -> Terminator6/1
  Demux/4 -> MATLAB Function4/2(yaw_des)
  MATLAB Function1/4(max_y_accel) -> Continuous Sigmoid1/3
  MATLAB Function/1(enable) -> Use desired X when enabled/Enable
  Continuous Sigmoid3/4 -> Terminator9/1
  MATLAB Function4/2(yaw_ref) -> Use des yaw when enabled/1(h_d (m) [1])
  FSM State (0,9)/1 -> Signmoid Type/1(FSM_state)
  MATLAB Function2/4(max_height_accel) -> Continuous Sigmoid2/3
  Continuous Sigmoid/4 -> Terminator3/1
  Continuous Sigmoid/3 -> Terminator2/1
  Continuous Sigmoid/1 -> MATLAB Function/5(x_cur)
  Continuous Sigmoid/2 -> MATLAB Function/6(x_vel)
  MATLAB Function/2(x_ref) -> Use desired X when enabled/1(h_d (m) [1])
  Continuous Sigmoid3/1 -> Mux2/4, MATLAB Function4/5(yaw_cur)
  MATLAB Function4/3(max_yaw_vel) -> Continuous Sigmoid3/2
  Continuous Sigmoid2/1 -> Mux2/3, MATLAB Function2/5(height_cur)
  Demux1/2 -> MATLAB Function1/7(y_meas)
  Constant3/1 -> MATLAB Function2/4(fast_lim)
  Continuous Sigmoid1/3 -> Terminator4/1
  "HF Measured Pose (m, rad) [4]"/1 -> Selector1/1, Demux1/1
  "HF Desired Pose (m, rad) [4]"/1 -> Selector2/1, Demux/1
  Use des height when enabled/1(Out1) -> Continuous Sigmoid2/1
  Use desired X when enabled/1(Out1) -> Mux2/1, Continuous Sigmoid/1

== system Commander_Stabilizer_Qdrone_serial/COMMANDER (PARALLEL CONTROL)/POSITION CONTROLLER (PARALLEL) ==
  note: X -> Pitch Torque
      | Y -> Roll Torque
      | Height -> Thrust Force
      | Yaw -> Yaw Torque
  note: 2
  note: 1
  note: 1. Generate a body frame pitch torque, roll torque, thrust and yaw torque output based on horizon frame position errors
      | 2. Remap controller output to the standard Generalized Force format (Thrust force, Roll torque, Pitch torque, Yaw torque).
  note: order: X, Y, Z, yaw
  note: PRTY to T(-R)PY
  note: PIV Controller
  note: Command Mapping
  note: Note that motion in X direction would warrant a positive pitch torque
      | and motion in the Y direction would require a negative roll torque
  "HF Pose Command (m, rad) [4]" : Inport
  "HF Pose Estimate (m, rad) [4]" : Inport  Port=2
  "HF Pose Rate (m/s, rad/s) [4]" : Inport  Port=3
  Reset : Inport  Port=4
  " " : Product  Multiplication=Matrix(*)
  Constant2 : Constant  Value=[0 0 1 0; 0 -1 0 0; 1 0 0 0; 0 0 0 1]
  Demux : Demux  Outputs=[2 2 2 2]
  Demux1 : Demux
  Integrator1 : Integrator  ExternalReset=rising  LimitOutput=on  UpperSaturationLimit=[0.26 0.33 5.825 0.05]  LowerSaturationLimit=[-0.26 -0.33 -5.825 -0.05]
  "Kd (N.m / m/s, N.m / m/s, N / m/s, Nm / rad/s)" : Gain  Gain=[0.55 .55 12 2]
  "Ki (N.m / m.s, N.m / m.s, N / m.s, N.m / rad.s)" : Gain  Gain=[0 0 3 0]
  "Kp (N.m / m, N.m / m, N / m, N.m / rad)" : Gain  Gain=[1.66 1.66 35 15]
  Mux : Mux  Inputs=2
  Note- Throttle is saturated to 80% of Trim Throttle : Saturate  UpperLimit=[pi/4 pi/4 35 10*pi/18]  LowerLimit=[-pi/4 -pi/4 -35 -10*pi/18]
  Position Tracking Performance (Horizontal Reference Frame) : Scope  NumInputPorts=4
  Selector : Selector  InputPortWidth=8  IndexOptions=Index vector (dialog)  Indices=[3 7 1 5 2 6 4 8]  OutputSizes=1
  Sum2 : Sum  Inputs=++-
  Sum3 : Sum  Inputs=|+-
  "Generalized Forces (N, Nm) [4]" : Outport
  tag scope: error_z=global
  wires:
  Reset/1 -> Integrator1/2
  "HF Pose Rate (m/s, rad/s) [4]"/1 -> "Kd (N.m / m/s, N.m / m/s, N / m/s, Nm / rad/s)"/1
  Mux/1 -> Selector/1
  Integrator1/1 -> Sum2/2
  "Ki (N.m / m.s, N.m / m.s, N / m.s, N.m / rad.s)"/1 -> Integrator1/1
  Selector/1 -> Demux/1
  " "/1 -> "Generalized Forces (N, Nm) [4]"/1
  Sum3/1 -> Demux1/1, "Ki (N.m / m.s, N.m / m.s, N / m.s, N.m / rad.s)"/1, "Kp (N.m / m, N.m / m, N / m, N.m / rad)"/1
  Note- Throttle is saturated to 80% of Trim Throttle/1 -> " "/2
  "HF Pose Estimate (m, rad) [4]"/1 -> Mux/2, Sum3/2
  Demux/1 -> Position Tracking Performance (Horizontal Reference Frame)/1
  "Kp (N.m / m, N.m / m, N / m, N.m / rad)"/1 -> Sum2/1
  Demux/2 -> Position Tracking Performance (Horizontal Reference Frame)/2
  "Kd (N.m / m/s, N.m / m/s, N / m/s, Nm / rad/s)"/1 -> Sum2/3
  Demux/3 -> Position Tracking Performance (Horizontal Reference Frame)/3
  Sum2/1 -> Note- Throttle is saturated to 80% of Trim Throttle/1
  "HF Pose Command (m, rad) [4]"/1 -> Sum3/1, Mux/1
  Demux/4 -> Position Tracking Performance (Horizontal Reference Frame)/4
  Constant2/1 -> " "/1
  Demux1/3 -> [error_z]

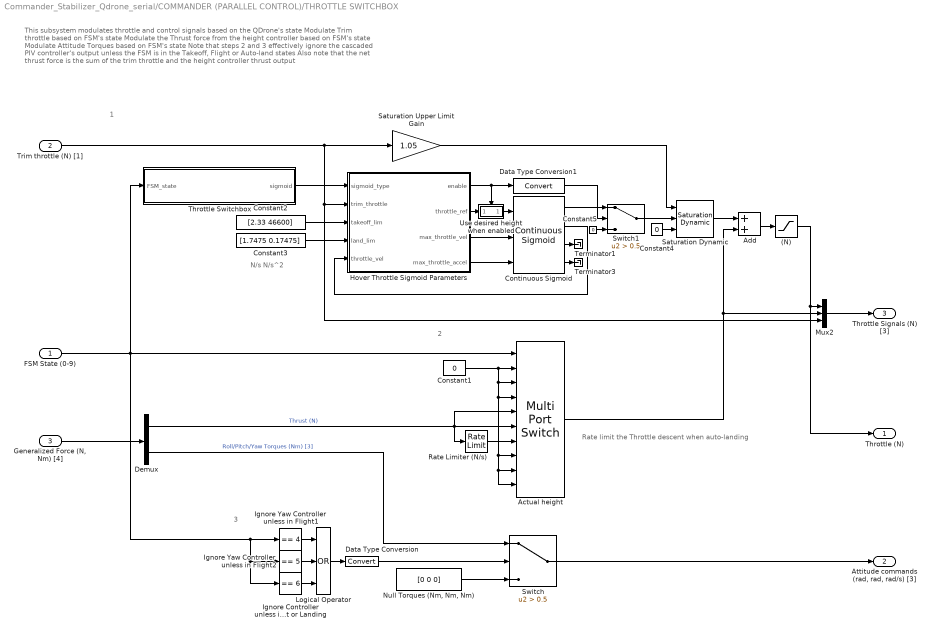
== system Commander_Stabilizer_Qdrone_serial/COMMANDER (PARALLEL CONTROL)/THROTTLE SWITCHBOX  ==
  note: 3
  note: 2
  note: 1
  note: Rate limit the Throttle descent when auto-landing
  note: This subsystem modulates throttle and control signals based on the QDrone's state
      | Modulate Trim throttle based on FSM's state
      | Modulate the Thrust force from the height controller based on FSM's state
      | Modulate Attitude Torques based on FSM's state
      |
      | Note that steps 2 and 3 effectively ignore the cascaded PIV controller's output unless the FSM is in the Takeoff, Flight or Auto-land states
      | Also note that the net thrust force is the sum of the trim throttle and the height controller thrust output
  note: N/s N/s^2
  FSM State (0-9) : Inport
  Trim throttle (N) [1] : Inport  Port=2
  "Generalized Force (N, Nm) [4]" : Inport  Port=3
  (N) : Saturate  UpperLimit=23.3  LowerLimit=0
  Actual height : MultiPortSwitch  Inputs=9
  Add : Sum
  Constant1 : Constant  Value=0
  Constant2 : Constant  Value=[2.33 46600]
  Constant3 : Constant  Value=[1.7475 0.17475]
  Constant4 : Constant  Value=0
  Constant5 : Constant  Value=0
  Continuous Sigmoid : quarc_library/Sources/Sigmoids/Continuous Sigmoid  params_source=External (input ports)  max_velocity=2  max_acceleration=10  initial_position=0  initial_velocity=0  hold_off=0.5  input_sample_time=-1  output_sample_time=qc_get_step_size
      settings: SourceProductName=QUARC Targets
  Data Type Conversion : DataTypeConversion
  Data Type Conversion1 : DataTypeConversion
  Demux : Demux  Outputs=[1 3]
  Hover Throttle Sigmoid Parameters : MATLAB Function  TreatAsAtomicUnit=on
  "Ignore Controller unless in Takeoff, Flight or Landing" : simulink/Logic and Bit Operations/Compare To Constant  relop===  const=6  OutDataTypeStr=boolean
  Ignore Yaw Controller unless in Flight1 : simulink/Logic and Bit Operations/Compare To Constant  relop===  const=4  OutDataTypeStr=boolean
  Ignore Yaw Controller unless in Flight2 : simulink/Logic and Bit Operations/Compare To Constant  relop===  const=5  OutDataTypeStr=boolean
  Logical Operator : Logic  Operator=OR  Inputs=3  AllPortsSameDT=off  OutDataTypeStr=boolean
  Mux2 : Mux  Inputs=3
  "Null Torques (Nm, Nm, Nm)" : Constant  Value=[0 0 0]
  Rate Limiter (N/s) : RateLimiter  RisingSlewLimit=100  FallingSlewLimit=-100  SampleTimeMode=inherited
  Saturation Dynamic : simulink/Discontinuities/Saturation Dynamic  OutMin=[]  OutMax=[]  OutDataTypeStr=Inherit: Same as second input  OutDataType=fixdt(1, 16)  OutScaling=2^-10  DoSatur=off
  Saturation Upper Limit Gain : Gain  Gain=1.05
  Switch : Switch  Criteria=u2 > Threshold  Threshold=0.5
  Switch1 : Switch  Criteria=u2 > Threshold  Threshold=0.5
  Terminator1 : Terminator
  Terminator3 : Terminator
  Throttle Switchbox : MATLAB Function  TreatAsAtomicUnit=on
  Use desired height when enabled : Subsystem  TreatAsAtomicUnit=on
  Throttle (N) : Outport
  "Attitude commands (rad, rad, rad/s) [3]" : Outport  Port=2
  Throttle Signals (N) [3] : Outport  Port=3
  wires:
  Actual height/1 -> Mux2/2, Add/2
  Add/1 -> (N)/1
  (N)/1 -> Mux2/1, Throttle (N)/1
  "Generalized Force (N, Nm) [4]"/1 -> Demux/1
  Mux2/1 -> Throttle Signals (N) [3]/1
  Ignore Yaw Controller unless in Flight2/1 -> Logical Operator/2
  Data Type Conversion/1 -> Switch/2
  "Null Torques (Nm, Nm, Nm)"/1 -> Switch/3
  Ignore Yaw Controller unless in Flight1/1 -> Logical Operator/1
  FSM State (0-9)/1 -> Actual height/1, "Ignore Controller unless in Takeoff, Flight or Landing"/1, Ignore Yaw Controller unless in Flight2/1, Ignore Yaw Controller unless in Flight1/1, Throttle Switchbox/1(FSM_state)
  "Ignore Controller unless in Takeoff, Flight or Landing"/1 -> Logical Operator/3
  Logical Operator/1 -> Data Type Conversion/1
  Demux/1 -> Rate Limiter (N/s)/1, Actual height/6, Actual height/5  "Thrust (N)"
  Continuous Sigmoid/2 -> Hover Throttle Sigmoid Parameters/5(throttle_vel)
  Constant4/1 -> Saturation Dynamic/3
  Saturation Dynamic/1 -> Add/1
  Constant3/1 -> Hover Throttle Sigmoid Parameters/4(land_lim)
  Switch1/1 -> Saturation Dynamic/2
  Trim throttle (N) [1]/1 -> Mux2/3, Hover Throttle Sigmoid Parameters/2(trim_throttle), Saturation Upper Limit Gain/1
  Throttle Switchbox/1(sigmoid) -> Hover Throttle Sigmoid Parameters/1(sigmoid_type)
  Saturation Upper Limit Gain/1 -> Saturation Dynamic/1
  Constant2/1 -> Hover Throttle Sigmoid Parameters/3(takeoff_lim)
  Hover Throttle Sigmoid Parameters/4(max_throttle_accel) -> Continuous Sigmoid/3
  Continuous Sigmoid/1 -> Switch1/1
  Continuous Sigmoid/4 -> Terminator3/1
  Hover Throttle Sigmoid Parameters/3(max_throttle_vel) -> Continuous Sigmoid/2
  Data Type Conversion1/1 -> Switch1/2
  Hover Throttle Sigmoid Parameters/1(enable) -> Data Type Conversion1/1, Use desired height when enabled/Enable
  Continuous Sigmoid/3 -> Terminator1/1
  Use desired height when enabled/1(Out1) -> Continuous Sigmoid/1
  Hover Throttle Sigmoid Parameters/2(throttle_ref) -> Use desired height when enabled/1(h_d (m) [1])
  Constant5/1 -> Switch1/3
  Switch/1 -> "Attitude commands (rad, rad, rad/s) [3]"/1
  Constant1/1 -> Actual height/8, Actual height/10, Actual height/9, Actual height/4, Actual height/3, Actual height/2
  Rate Limiter (N/s)/1 -> Actual height/7
  Demux/2 -> Switch/1  "Roll/Pitch/Yaw Torques (Nm) [3]"

== system Commander_Stabilizer_Qdrone_serial/Communication/Detect Communication Loss ==
  note: Check if the state is 2 and error is positive (error codes are negative). Otherwise issue a communication error.
      | OR
      | Check if the data is stale for a while (this is required because a connected stream may publish no new data). If stale, issue a communication error.
  State : Inport
  Error : Inport  Port=2
  Data Out : Inport  Port=3
  Clock1 : Clock
  Data Type Conversion4 : DataTypeConversion
  Grab height measurement to detect flat lines : Selector  InputPortWidth=15  IndexOptions=Index vector (dialog)  Indices=[7]  OutputSizes=1
  Logical Operator4 : Logic  Operator=OR  AllPortsSameDT=off  OutDataTypeStr=boolean
  MATLAB Function : MATLAB Function  TreatAsAtomicUnit=on
  Maximum height while on ground (cm) : Constant  Value=0.05
  Terminator3 : Terminator
  Terminator5 : Terminator
  Threshold1 : quarc_library/Discontinuities/Threshold  operator=>=  param_src=Specify via dialog  threshold=0.5  duration=0.1
      settings: SourceProductName=QUARC Targets
  Threshold2 : quarc_library/Discontinuities/Threshold  operator=>=  param_src=Specify via dialog  threshold=0.5  duration=0.5
      settings: SourceProductName=QUARC Targets
  Communication Issue : Outport
  wires:
  Threshold2/1 -> Logical Operator4/2
  Logical Operator4/1 -> Data Type Conversion4/1
  Threshold1/2 -> Terminator3/1
  MATLAB Function/2(data_loss) -> Threshold2/1
  MATLAB Function/1(stream_connection_loss) -> Threshold1/1
  Clock1/1 -> MATLAB Function/1(time)
  Threshold2/2 -> Terminator5/1
  Threshold1/1 -> Logical Operator4/1
  Grab height measurement to detect flat lines/1 -> MATLAB Function/4(height)
  Data Out/1 -> Grab height measurement to detect flat lines/1
  State/1 -> MATLAB Function/2(state)
  Error/1 -> MATLAB Function/3(error)
  Data Type Conversion4/1 -> Communication Issue/1
  Maximum height while on ground (cm)/1 -> MATLAB Function/5(minimum_flight_height)

== system Commander_Stabilizer_Qdrone_serial/HORIZON FRAME CONVERSION AND ESTIMATION/Calculate Rotation Matrices ==
  note: Generate rotation matrices:
      | A_R_B is a rotation matrix FROM frame B TO frame A.
  " Roll Estimate (rad)" : Inport
  Pitch Estimate (rad) : Inport  Port=2
  Yaw Estimate (rad) : Inport  Port=3
  MATLAB Function2 : MATLAB Function  TreatAsAtomicUnit=on
  MATLAB Function4 : MATLAB Function  TreatAsAtomicUnit=on
  HF_R_BF : Outport
  HF_R_IF : Outport  Port=2
  wires:
  " Roll Estimate (rad)"/1 -> MATLAB Function2/1(roll)
  Yaw Estimate (rad)/1 -> MATLAB Function4/1(yaw)
  Pitch Estimate (rad)/1 -> MATLAB Function2/2(pitch)
  MATLAB Function4/1(HF_R_IF) -> HF_R_IF/1
  MATLAB Function2/1(HF_R_BF) -> HF_R_BF/1
